simulink model "Channelizer_hil"  (R2023b)
settings: Solver=VariableStepAuto  StartTime=0.0  StopTime=inf  RelTol=1e-3
InitFcn:
  | init
values from neighbouring files (symbols this model uses):
  N = 2*1024    (= 2048)    [hil.m]    (also in init.m)
undefined symbols (not defined in the file or in its folder): ch0, ch1, ch10, ch11, ch12, ch13, ch14, ch15, ch2, ch3, ch4, ch5, ch6, ch7, ch8, ch9, S, vsva2197, xcvc1902
libraries: aieUtilities x47, aieBasic x34, hlsBasic x3, dspindex x3, vmcUtilities x1, commchan3 x1, commrflib2 x1, commfilt2 x1, commrandsrc3 x1, commdigbbndam3 x1
(part 2 of 2)

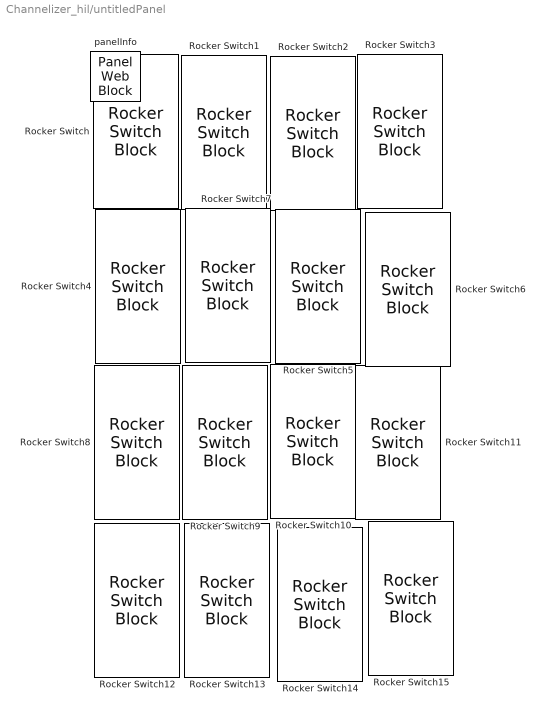
== system Channelizer_hil/untitledPanel ==
  Rocker Switch : RockerSwitchBlock  Tag=HiddenForWebPanel  PanelInfo="{\"addnFilesFolder\":\"\",\"height\":154,\"includeDebugPackages\":false,\"left\":10,\"outputFolder\":\"\",\"panelId\":\"panelId-fec1c322-f5e7-4e4f-8c31-b98d6132c1cd\",\"popoutMode\":\"\",\"standaloneTitle\":\"\",\"top\":12,\"type\":\"panelChild\",\"version\":\"2019b\",\"width\":85,\"zIndex\":1500002}"
      settings: Values={{'Off', 'On'}, [0 1]}
  Rocker Switch1 : RockerSwitchBlock  Tag=HiddenForWebPanel  PanelInfo="{\"addnFilesFolder\":\"\",\"height\":154,\"includeDebugPackages\":false,\"left\":98,\"outputFolder\":\"\",\"panelId\":\"panelId-fec1c322-f5e7-4e4f-8c31-b98d6132c1cd\",\"popoutMode\":\"\",\"standaloneTitle\":\"\",\"top\":12,\"type\":\"panelChild\",\"version\":\"2019b\",\"width\":85,\"zIndex\":1500004}"
      settings: Values={{'Off', 'On'}, [0 1]}
  Rocker Switch10 : RockerSwitchBlock  Tag=HiddenForWebPanel  PanelInfo="{\"addnFilesFolder\":\"\",\"height\":154,\"includeDebugPackages\":false,\"left\":185,\"outputFolder\":\"\",\"panelId\":\"panelId-fec1c322-f5e7-4e4f-8c31-b98d6132c1cd\",\"popoutMode\":\"\",\"standaloneTitle\":\"\",\"top\":327,\"type\":\"panelChild\",\"version\":\"2019b\",\"width\":85,\"zIndex\":1500022}"
      settings: Values={{'Off', 'On'}, [0 1]}
  Rocker Switch11 : RockerSwitchBlock  Tag=HiddenForWebPanel  PanelInfo="{\"addnFilesFolder\":\"\",\"height\":154,\"includeDebugPackages\":false,\"left\":273,\"outputFolder\":\"\",\"panelId\":\"panelId-fec1c322-f5e7-4e4f-8c31-b98d6132c1cd\",\"popoutMode\":\"\",\"standaloneTitle\":\"\",\"top\":327,\"type\":\"panelChild\",\"version\":\"2019b\",\"width\":85,\"zIndex\":1500024}"
      settings: Values={{'Off', 'On'}, [0 1]}
  Rocker Switch12 : RockerSwitchBlock  Tag=HiddenForWebPanel  PanelInfo="{\"addnFilesFolder\":\"\",\"height\":154,\"includeDebugPackages\":false,\"left\":10,\"outputFolder\":\"\",\"panelId\":\"panelId-fec1c322-f5e7-4e4f-8c31-b98d6132c1cd\",\"popoutMode\":\"\",\"standaloneTitle\":\"\",\"top\":483,\"type\":\"panelChild\",\"version\":\"2019b\",\"width\":85,\"zIndex\":1500026}"
      settings: Values={{'Off', 'On'}, [0 1]}
  Rocker Switch13 : RockerSwitchBlock  Tag=HiddenForWebPanel  PanelInfo="{\"addnFilesFolder\":\"\",\"height\":154,\"includeDebugPackages\":false,\"left\":97,\"outputFolder\":\"\",\"panelId\":\"panelId-fec1c322-f5e7-4e4f-8c31-b98d6132c1cd\",\"popoutMode\":\"\",\"standaloneTitle\":\"\",\"top\":483,\"type\":\"panelChild\",\"version\":\"2019b\",\"width\":85,\"zIndex\":1500028}"
      settings: Values={{'Off', 'On'}, [0 1]}
  Rocker Switch14 : RockerSwitchBlock  Tag=HiddenForWebPanel  PanelInfo="{\"addnFilesFolder\":\"\",\"height\":154,\"includeDebugPackages\":false,\"left\":185,\"outputFolder\":\"\",\"panelId\":\"panelId-fec1c322-f5e7-4e4f-8c31-b98d6132c1cd\",\"popoutMode\":\"\",\"standaloneTitle\":\"\",\"top\":484,\"type\":\"panelChild\",\"version\":\"2019b\",\"width\":85,\"zIndex\":1500030}"
      settings: Values={{'Off', 'On'}, [0 1]}
  Rocker Switch15 : RockerSwitchBlock  Tag=HiddenForWebPanel  PanelInfo="{\"addnFilesFolder\":\"\",\"height\":154,\"includeDebugPackages\":false,\"left\":272,\"outputFolder\":\"\",\"panelId\":\"panelId-fec1c322-f5e7-4e4f-8c31-b98d6132c1cd\",\"popoutMode\":\"\",\"standaloneTitle\":\"\",\"top\":484,\"type\":\"panelChild\",\"version\":\"2019b\",\"width\":85,\"zIndex\":1500032}"
      settings: Values={{'Off', 'On'}, [0 1]}
  Rocker Switch2 : RockerSwitchBlock  Tag=HiddenForWebPanel  PanelInfo="{\"addnFilesFolder\":\"\",\"height\":154,\"includeDebugPackages\":false,\"left\":186,\"outputFolder\":\"\",\"panelId\":\"panelId-fec1c322-f5e7-4e4f-8c31-b98d6132c1cd\",\"popoutMode\":\"\",\"standaloneTitle\":\"\",\"top\":12,\"type\":\"panelChild\",\"version\":\"2019b\",\"width\":85,\"zIndex\":1500006}"
      settings: Values={{'Off', 'On'}, [0 1]}
  Rocker Switch3 : RockerSwitchBlock  Tag=HiddenForWebPanel  PanelInfo="{\"addnFilesFolder\":\"\",\"height\":154,\"includeDebugPackages\":false,\"left\":274,\"outputFolder\":\"\",\"panelId\":\"panelId-fec1c322-f5e7-4e4f-8c31-b98d6132c1cd\",\"popoutMode\":\"\",\"standaloneTitle\":\"\",\"top\":12,\"type\":\"panelChild\",\"version\":\"2019b\",\"width\":85,\"zIndex\":1500008}"
      settings: Values={{'Off', 'On'}, [0 1]}
  Rocker Switch4 : RockerSwitchBlock  Tag=HiddenForWebPanel  PanelInfo="{\"addnFilesFolder\":\"\",\"height\":154,\"includeDebugPackages\":false,\"left\":10,\"outputFolder\":\"\",\"panelId\":\"panelId-fec1c322-f5e7-4e4f-8c31-b98d6132c1cd\",\"popoutMode\":\"\",\"standaloneTitle\":\"\",\"top\":169,\"type\":\"panelChild\",\"version\":\"2019b\",\"width\":85,\"zIndex\":1500010}"
      settings: Values={{'Off', 'On'}, [0 1]}
  Rocker Switch5 : RockerSwitchBlock  Tag=HiddenForWebPanel  PanelInfo="{\"addnFilesFolder\":\"\",\"height\":154,\"includeDebugPackages\":false,\"left\":186,\"outputFolder\":\"\",\"panelId\":\"panelId-fec1c322-f5e7-4e4f-8c31-b98d6132c1cd\",\"popoutMode\":\"\",\"standaloneTitle\":\"\",\"top\":170,\"type\":\"panelChild\",\"version\":\"2019b\",\"width\":85,\"zIndex\":1500012}"
      settings: Values={{'Off', 'On'}, [0 1]}
  Rocker Switch6 : RockerSwitchBlock  Tag=HiddenForWebPanel  PanelInfo="{\"addnFilesFolder\":\"\",\"height\":154,\"includeDebugPackages\":false,\"left\":274,\"outputFolder\":\"\",\"panelId\":\"panelId-fec1c322-f5e7-4e4f-8c31-b98d6132c1cd\",\"popoutMode\":\"\",\"standaloneTitle\":\"\",\"top\":170,\"type\":\"panelChild\",\"version\":\"2019b\",\"width\":85,\"zIndex\":1500014}"
      settings: Values={{'Off', 'On'}, [0 1]}
  Rocker Switch7 : RockerSwitchBlock  Tag=HiddenForWebPanel  PanelInfo="{\"addnFilesFolder\":\"\",\"height\":154,\"includeDebugPackages\":false,\"left\":98,\"outputFolder\":\"\",\"panelId\":\"panelId-fec1c322-f5e7-4e4f-8c31-b98d6132c1cd\",\"popoutMode\":\"\",\"standaloneTitle\":\"\",\"top\":169,\"type\":\"panelChild\",\"version\":\"2019b\",\"width\":85,\"zIndex\":1500016}"
      settings: Values={{'Off', 'On'}, [0 1]}
  Rocker Switch8 : RockerSwitchBlock  Tag=HiddenForWebPanel  PanelInfo="{\"addnFilesFolder\":\"\",\"height\":154,\"includeDebugPackages\":false,\"left\":10,\"outputFolder\":\"\",\"panelId\":\"panelId-fec1c322-f5e7-4e4f-8c31-b98d6132c1cd\",\"popoutMode\":\"\",\"standaloneTitle\":\"\",\"top\":326,\"type\":\"panelChild\",\"version\":\"2019b\",\"width\":85,\"zIndex\":1500018}"
      settings: Values={{'Off', 'On'}, [0 1]}
  Rocker Switch9 : RockerSwitchBlock  Tag=HiddenForWebPanel  PanelInfo="{\"addnFilesFolder\":\"\",\"height\":154,\"includeDebugPackages\":false,\"left\":97,\"outputFolder\":\"\",\"panelId\":\"panelId-fec1c322-f5e7-4e4f-8c31-b98d6132c1cd\",\"popoutMode\":\"\",\"standaloneTitle\":\"\",\"top\":326,\"type\":\"panelChild\",\"version\":\"2019b\",\"width\":85,\"zIndex\":1500020}"
      settings: Values={{'Off', 'On'}, [0 1]}
  panelInfo : PanelWebBlock  Tag=HiddenForWebPanel  PanelInfo="{\"addnFilesFolder\":\"\",\"compacted\":false,\"height\":655,\"includeDebugPackages\":false,\"isActiveTab\":true,\"left\":-4,\"name\":\"Panel\",\"outputFolder\":\"\",\"panelId\":\"panelId-fec1c322-f5e7-4e4f-8c31-b98d6132c1cd\",\"popoutMode\":\"\",\"standaloneTitle\":\"\",\"tabIndex\":0,\"tabbedSetId\":\"tabbedSet6868322055\",\"top\":96,\"type\":\"panel\",\"version\":\"2019b\",\"visible\":true,\"width\":371,\"zIndex\":1500002}"  PanelSnapshot=<binary blob, 10492 chars, not shown>

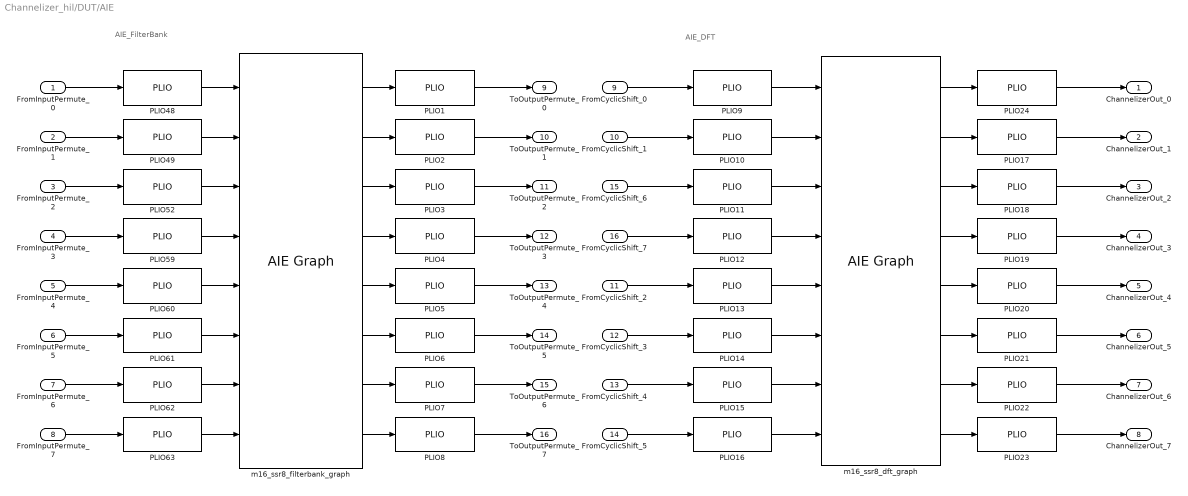
== system Channelizer_hil/DUT/AIE ==
  note: AIE_DFT
  note: AIE_FilterBank
  FromInputPermute_0 : Inport
  FromInputPermute_1 : Inport  Port=2
  FromInputPermute_2 : Inport  Port=3
  FromInputPermute_3 : Inport  Port=4
  FromInputPermute_4 : Inport  Port=5
  FromInputPermute_5 : Inport  Port=6
  FromInputPermute_6 : Inport  Port=7
  FromInputPermute_7 : Inport  Port=8
  FromCyclicShift_0 : Inport  Port=9
  FromCyclicShift_1 : Inport  Port=10
  FromCyclicShift_2 : Inport  Port=11
  FromCyclicShift_3 : Inport  Port=12
  FromCyclicShift_4 : Inport  Port=13
  FromCyclicShift_5 : Inport  Port=14
  FromCyclicShift_6 : Inport  Port=15
  FromCyclicShift_7 : Inport  Port=16
  PLIO{1..24,48..49,52,59..63} (32 alike) : aieBasic/PLIO  PlioWidth=64  PlioFreqSpec=on  PlioFreq=625  ColLocation=0  channel=0  blockJsonConstraints=[]  deprecateConstraints=0
  m16_ssr8_dft_graph : aieBasic/AIE Graph  PortAttributesTable={ 'Input', 'sig_i[0]', 'stream', 'cint16', '', '', ''; 'Input', 'sig_i[1]', 'stream', 'cint16', '', '', ''; 'Input', 'sig_i[6]', 'stream', 'cint16', '', '', ''; 'Input', 'sig_i[7]', 'stream', 'cint16', '', '', ''; 'Input', 'sig_i[2]', 'stream', 'cint16', '', '', ''; 'Input', 'sig_i[3]', 'stream', 'cint16', '', '', ''; 'Input', 'sig_i[4]', 'stream', 'cint16', '', '', ''; 'Input', 'sig_i[5]', 'stream', 'cint16', '', '', ''; 'Output', 'sig_o[0]', 'stream', 'cint16', '', '', '4*N'; 'Output', 'sig_o[1]', 'stream', 'cint16', '', '', '4*N'; 'Output', 'sig_o[2]', 'stream', 'cint16', '', '', '4*N'; 'Output', 'sig_o[3]', 'stream', 'cint16', '', '', '4*N'; 'Output', 'sig_o[4]', 'stream', 'cint16', '', '', '4*N'; 'Output', 'sig_o[5]', 'stream', 'cint16', '', '', '4*N'; 'Output', 'sig_o[6]', 'stream', 'cint16', '', '', '4*N'; 'Output', 'sig_o[7]', 'stream', 'cint16', '', '', '4*N' }  PortAttributesEnablement={'off', 'on', 'off', 'off', 'off', 'off', 'off';'off', 'on', 'off', 'off', 'off', 'off', 'off';'off', 'on', 'off', 'off', 'off', 'off', 'off';'off', 'on', 'off', 'off', 'off', 'off', 'off';'off', 'on', 'off', 'off', 'off', 'off', 'off';'off', 'on', 'off', 'off', 'off', 'off', 'off';'off', 'on', 'off', 'off', 'off', 'off', 'off';'off', 'on', 'off', 'off', 'off', 'off', 'off';'off', 'on', 'off', 'off', 'off', 'off', 'on';'off', 'on', 'off', 'off', 'off', 'off', 'on';'off', 'on', 'off', 'off', 'off', 'off', 'on';'off', 'on', 'off', 'off', 'off', 'off', 'on';'off', 'on', 'off', 'off', 'off', 'off', 'on';'off', 'on', 'off', 'off', 'off', 'off', 'on';'off', 'on', 'off', 'off', 'off', 'off', 'on';'off', 'on', 'off', 'off', 'off', 'off', 'on'}  SampleTime=-1  ClassDeclTypeOptions=C[1 1]@t24@class m16_ssr8_dft_graph  ClassDecl=class m16_ssr8_dft_graph  ClassTemplateParams={}  ClassTemplateParamsEnables={}  ClassCtorDeclTypeOptions=C[1 1]@t7@<empty>  ClassCtorDecl=<empty>  ClassCtorParams={}  GraphAllAttrs=|  PortArgDecls={'in stream cint16 in1'; 'in stream cint16 in2'; 'in stream cint16 in3'; 'in stream cint16 in4'; 'in stream cint16 in5'; 'in stream cint16 in6'; 'in stream cint16 in7'; 'in stream cint16 in8'; 'out stream cint16 out1'; 'out stream cint16 out2'; 'out stream cint16 out3'; 'out stream cint16 out4'; 'out stream cint16 out5'; 'out stream cint16 out6'; 'out stream cint16 out7'; 'out stream cint16 out8'}  PortGraphPortNames={'sig_i[0]'; 'sig_i[1]'; 'sig_i[6]'; 'sig_i[7]'; 'sig_i[2]'; 'sig_i[3]'; 'sig_i[4]'; 'sig_i[5]'; 'sig_o[0]'; 'sig_o[1]'; 'sig_o[2]'; 'sig_o[3]'; 'sig_o[4]'; 'sig_o[5]'; 'sig_o[6]'; 'sig_o[7]'}  PortTypes={'stream'; 'stream'; 'stream'; 'stream'; 'stream'; 'stream'; 'stream'; 'stream'; 'stream'; 'stream'; 'stream'; 'stream'; 'stream'; 'stream'; 'stream'; 'stream'}  PortDataTypes={'cint16'; 'cint16'; 'cint16'; 'cint16'; 'cint16'; 'cint16'; 'cint16'; 'cint16'; 'cint16'; 'cint16'; 'cint16'; 'cint16'; 'cint16'; 'cint16'; 'cint16'; 'cint16'}  PortSizes={0.000000000000000000e+00; 0.000000000000000000e+00; 0.000000000000000000e+00; 0.000000000000000000e+00; 0.000000000000000000e+00; 0.000000000000000000e+00; 0.000000000000000000e+00; 0.000000000000000000e+00; 0.000000000000000000e+00; 0.000000000000000000e+00; 0.000000000000000000e+00; 0.000000000000000000e+00; 0.000000000000000000e+00; 0.000000000000000000e+00; 0.000000000000000000e+00; 0.000000000000000000e+00}  PortSynchronicities={'auto'; 'auto'; 'auto'; 'auto'; 'auto'; 'auto'; 'auto'; 'auto'; 'auto'; 'auto'; 'auto'; 'auto'; 'auto'; 'auto'; 'auto'; 'auto'}  PortSignalSizes={0.000000000000000000e+00; 0.000000000000000000e+00; 0.000000000000000000e+00; 0.000000000000000000e+00; 0.000000000000000000e+00; 0.000000000000000000e+00; 0.000000000000000000e+00; 0.000000000000000000e+00; 8.192000000000000000e+03; 8.192000000000000000e+03; 8.192000000000000000e+03; 8.192000000000000000e+03; 8.192000000000000000e+03; 8.192000000000000000e+03; 8.192000000000000000e+03; 8.192000000000000000e+03}  SimLibPath=''  ClassIndex=1  ClassCtorIndex=0  ClassTabVisible=off  FunctionTabVisible=on  DelayDrawLabels=off  GraphFileSelect=Header file (*.h)  GraphHeaderFile=./aie/m16_ssr8_dft_graph.h  GraphClassName=m16_ssr8_dft_graph  GraphName=m16_ssr8_dft_graph  GraphHeaderFiles={'./aie/dft_1xN_widget_graph.h'; './aie/m16_ssr8_dft_graph.h'}  GraphSourceFile=./model_composer_work/xmc_aie_lib/8d40d72d/mygraph.cpp  GraphSearchPaths={'./aie'}  GraphPreProcOptions={}  blockJsonConstraints=[]
      | s[12;12;9;9;19;14;21;23;21;23;24;21;15;17;12;24;26;26;26;27;28;9;21;23;23;23;24;25;14;19;19;29]@FunctionNameDeclFileNamePortNamesPortTypesPortSerializedTypesPortDirectionsPortWindowSizeEnablesPortWindowMarginEnablesPortBufferSizeEnablesPortBufferMarginEnablesPortSynchronicityEnablesPortSignalSizeEnablesPortBufferSizesPortBufferMarginsFunctionDeclFunctionTemplateSpecKindFunctionTemplateParamNamesFunctionTemplateParamKindsFunctionTemplateParamTypesFunctionTemplateParamValuesFunctionTemplateParamEnablesClassDeclClassTemplateSpecKindClassTemplateParamNamesClassTemplateParamKindsClassTemplateParamTypesClassTemplateParamValuesClassTemplateParamEnablesClassCtorDeclsClassCtorParamNamesClassCtorParamTypesClassCtorParamSerializedTypes[1 1]@C[32 1]@nt30@../../aie/m16_ssr8_dft_graph.hC[2 1]@t5@sig_it5@sig_oC[2 1]@t48@std::array< adf::port< adf::direction::in >, 8 >t49@std::array< adf::port< adf::direction::out >, 8 >C[2 1]@t64@{Tstd::array{2{t{Tadf::port{1{t{Sadf::direction::in}}}}}{t{}8}}}t65@{Tstd::array{2{t{Tadf::port{1{t{Sadf::direction::out}}}}}{t{}8}}}C[2 1]@t5@inputt5@inputC[2 1]@l0@l0@C[2 1]@l0@l0@C[2 1]@l0@l0@C[2 1]@l0@l0@C[2 1]@l1@l1@C[2 1]@l0@l0@C[2 1]@nnC[2 1]@nnt139@void m16_ssr8_dft_graph::
      | (std::array< adf::port< adf::direction::in >, 8 > sig_i, std::array< adf::port< adf::direction::out >, 8 > sig_o)ne[0 1]@e[0 1]@e[0 1]@e[0 1]@e[0 1]@t25@class m16_ssr8_dft_graph;t4@nonee[0 1]@e[0 1]@e[0 1]@e[0 1]@e[0 1]@e[0 1]@e[0 1]@e[0 1]@e[0 1]@
  m16_ssr8_filterbank_graph : aieBasic/AIE Graph  PortAttributesTable={ 'Input', 'sig_i[0]', 'stream', 'cint16', '', '', ''; 'Input', 'sig_i[1]', 'stream', 'cint16', '', '', ''; 'Input', 'sig_i[2]', 'stream', 'cint16', '', '', ''; 'Input', 'sig_i[3]', 'stream', 'cint16', '', '', ''; 'Input', 'sig_i[4]', 'stream', 'cint16', '', '', ''; 'Input', 'sig_i[5]', 'stream', 'cint16', '', '', ''; 'Input', 'sig_i[6]', 'stream', 'cint16', '', '', ''; 'Input', 'sig_i[7]', 'stream', 'cint16', '', '', ''; 'Output', 'sig_o[0]', 'stream', 'cint16', '', '', '4*N'; 'Output', 'sig_o[1]', 'stream', 'cint16', '', '', '4*N'; 'Output', 'sig_o[2]', 'stream', 'cint16', '', '', '4*N'; 'Output', 'sig_o[3]', 'stream', 'cint16', '', '', '4*N'; 'Output', 'sig_o[4]', 'stream', 'cint16', '', '', '4*N'; 'Output', 'sig_o[5]', 'stream', 'cint16', '', '', '4*N'; 'Output', 'sig_o[6]', 'stream', 'cint16', '', '', '4*N'; 'Output', 'sig_o[7]', 'stream', 'cint16', '', '', '4*N' }  PortAttributesEnablement={'off', 'on', 'off', 'off', 'off', 'off', 'off';'off', 'on', 'off', 'off', 'off', 'off', 'off';'off', 'on', 'off', 'off', 'off', 'off', 'off';'off', 'on', 'off', 'off', 'off', 'off', 'off';'off', 'on', 'off', 'off', 'off', 'off', 'off';'off', 'on', 'off', 'off', 'off', 'off', 'off';'off', 'on', 'off', 'off', 'off', 'off', 'off';'off', 'on', 'off', 'off', 'off', 'off', 'off';'off', 'on', 'off', 'off', 'off', 'off', 'on';'off', 'on', 'off', 'off', 'off', 'off', 'on';'off', 'on', 'off', 'off', 'off', 'off', 'on';'off', 'on', 'off', 'off', 'off', 'off', 'on';'off', 'on', 'off', 'off', 'off', 'off', 'on';'off', 'on', 'off', 'off', 'off', 'off', 'on';'off', 'on', 'off', 'off', 'off', 'off', 'on';'off', 'on', 'off', 'off', 'off', 'off', 'on'}  SampleTime=-1  ClassDeclTypeOptions=C[1 1]@t31@class m16_ssr8_filterbank_graph  ClassDecl=class m16_ssr8_filterbank_graph  ClassTemplateParams={}  ClassTemplateParamsEnables={}  ClassCtorDeclTypeOptions=C[1 1]@t7@<empty>  ClassCtorDecl=<empty>  ClassCtorParams={}  GraphAllAttrs=|  PortArgDecls={'in stream cint16 in1'; 'in stream cint16 in2'; 'in stream cint16 in3'; 'in stream cint16 in4'; 'in stream cint16 in5'; 'in stream cint16 in6'; 'in stream cint16 in7'; 'in stream cint16 in8'; 'out stream cint16 out1'; 'out stream cint16 out2'; 'out stream cint16 out3'; 'out stream cint16 out4'; 'out stream cint16 out5'; 'out stream cint16 out6'; 'out stream cint16 out7'; 'out stream cint16 out8'}  PortGraphPortNames={'sig_i[0]'; 'sig_i[1]'; 'sig_i[2]'; 'sig_i[3]'; 'sig_i[4]'; 'sig_i[5]'; 'sig_i[6]'; 'sig_i[7]'; 'sig_o[0]'; 'sig_o[1]'; 'sig_o[2]'; 'sig_o[3]'; 'sig_o[4]'; 'sig_o[5]'; 'sig_o[6]'; 'sig_o[7]'}  PortTypes={'stream'; 'stream'; 'stream'; 'stream'; 'stream'; 'stream'; 'stream'; 'stream'; 'stream'; 'stream'; 'stream'; 'stream'; 'stream'; 'stream'; 'stream'; 'stream'}  PortDataTypes={'cint16'; 'cint16'; 'cint16'; 'cint16'; 'cint16'; 'cint16'; 'cint16'; 'cint16'; 'cint16'; 'cint16'; 'cint16'; 'cint16'; 'cint16'; 'cint16'; 'cint16'; 'cint16'}  PortSizes={0.000000000000000000e+00; 0.000000000000000000e+00; 0.000000000000000000e+00; 0.000000000000000000e+00; 0.000000000000000000e+00; 0.000000000000000000e+00; 0.000000000000000000e+00; 0.000000000000000000e+00; 0.000000000000000000e+00; 0.000000000000000000e+00; 0.000000000000000000e+00; 0.000000000000000000e+00; 0.000000000000000000e+00; 0.000000000000000000e+00; 0.000000000000000000e+00; 0.000000000000000000e+00}  PortSynchronicities={'auto'; 'auto'; 'auto'; 'auto'; 'auto'; 'auto'; 'auto'; 'auto'; 'auto'; 'auto'; 'auto'; 'auto'; 'auto'; 'auto'; 'auto'; 'auto'}  PortSignalSizes={0.000000000000000000e+00; 0.000000000000000000e+00; 0.000000000000000000e+00; 0.000000000000000000e+00; 0.000000000000000000e+00; 0.000000000000000000e+00; 0.000000000000000000e+00; 0.000000000000000000e+00; 8.192000000000000000e+03; 8.192000000000000000e+03; 8.192000000000000000e+03; 8.192000000000000000e+03; 8.192000000000000000e+03; 8.192000000000000000e+03; 8.192000000000000000e+03; 8.192000000000000000e+03}  SimLibPath=''  ClassIndex=1  ClassCtorIndex=0  ClassTabVisible=off  FunctionTabVisible=on  DelayDrawLabels=off  GraphFileSelect=Header file (*.h)  GraphHeaderFile=./aie/m16_ssr8_filterbank_graph.h  GraphClassName=m16_ssr8_filterbank_graph  GraphName=m16_ssr8_filterbank_graph  GraphHeaderFiles={'./aie/polyphase_fir_graph.h'; './aie/m16_ssr8_filterbank_graph.h'}  GraphSourceFile=./model_composer_work/xmc_aie_lib/fadd8e47/mygraph.cpp  GraphSearchPaths={'./aie'}  GraphPreProcOptions={}  blockJsonConstraints=[]
      | s[12;12;9;9;19;14;21;23;21;23;24;21;15;17;12;24;26;26;26;27;28;9;21;23;23;23;24;25;14;19;19;29]@FunctionNameDeclFileNamePortNamesPortTypesPortSerializedTypesPortDirectionsPortWindowSizeEnablesPortWindowMarginEnablesPortBufferSizeEnablesPortBufferMarginEnablesPortSynchronicityEnablesPortSignalSizeEnablesPortBufferSizesPortBufferMarginsFunctionDeclFunctionTemplateSpecKindFunctionTemplateParamNamesFunctionTemplateParamKindsFunctionTemplateParamTypesFunctionTemplateParamValuesFunctionTemplateParamEnablesClassDeclClassTemplateSpecKindClassTemplateParamNamesClassTemplateParamKindsClassTemplateParamTypesClassTemplateParamValuesClassTemplateParamEnablesClassCtorDeclsClassCtorParamNamesClassCtorParamTypesClassCtorParamSerializedTypes[1 1]@C[32 1]@nt37@../../aie/m16_ssr8_filterbank_graph.hC[2 1]@t5@sig_it5@sig_oC[2 1]@t48@std::array< adf::port< adf::direction::in >, 8 >t49@std::array< adf::port< adf::direction::out >, 8 >C[2 1]@t64@{Tstd::array{2{t{Tadf::port{1{t{Sadf::direction::in}}}}}{t{}8}}}t65@{Tstd::array{2{t{Tadf::port{1{t{Sadf::direction::out}}}}}{t{}8}}}C[2 1]@t5@inputt5@inputC[2 1]@l0@l0@C[2 1]@l0@l0@C[2 1]@l0@l0@C[2 1]@l0@l0@C[2 1]@l1@l1@C[2 1]@l0@l0@C[2 1]@nnC[2 1]@nnt146@void m16_ssr8_filterbank_graph::
      | (std::array< adf::port< adf::direction::in >, 8 > sig_i, std::array< adf::port< adf::direction::out >, 8 > sig_o)ne[0 1]@e[0 1]@e[0 1]@e[0 1]@e[0 1]@t32@class m16_ssr8_filterbank_graph;t4@nonee[0 1]@e[0 1]@e[0 1]@e[0 1]@e[0 1]@e[0 1]@e[0 1]@e[0 1]@e[0 1]@
  ChannelizerOut_0 : Outport
  ChannelizerOut_1 : Outport  Port=2
  ChannelizerOut_2 : Outport  Port=3
  ChannelizerOut_3 : Outport  Port=4
  ChannelizerOut_4 : Outport  Port=5
  ChannelizerOut_5 : Outport  Port=6
  ChannelizerOut_6 : Outport  Port=7
  ChannelizerOut_7 : Outport  Port=8
  ToOutputPermute_0 : Outport  Port=9
  ToOutputPermute_1 : Outport  Port=10
  ToOutputPermute_2 : Outport  Port=11
  ToOutputPermute_3 : Outport  Port=12
  ToOutputPermute_4 : Outport  Port=13
  ToOutputPermute_5 : Outport  Port=14
  ToOutputPermute_6 : Outport  Port=15
  ToOutputPermute_7 : Outport  Port=16
  wires:
  PLIO4/1 -> ToOutputPermute_3/1
  PLIO1/1 -> ToOutputPermute_0/1
  PLIO2/1 -> ToOutputPermute_1/1
  PLIO8/1 -> ToOutputPermute_7/1
  PLIO7/1 -> ToOutputPermute_6/1
  PLIO5/1 -> ToOutputPermute_4/1
  PLIO6/1 -> ToOutputPermute_5/1
  PLIO3/1 -> ToOutputPermute_2/1
  PLIO22/1 -> ChannelizerOut_6/1
  PLIO21/1 -> ChannelizerOut_5/1
  PLIO24/1 -> ChannelizerOut_0/1
  PLIO17/1 -> ChannelizerOut_1/1
  PLIO18/1 -> ChannelizerOut_2/1
  PLIO19/1 -> ChannelizerOut_3/1
  PLIO20/1 -> ChannelizerOut_4/1
  PLIO23/1 -> ChannelizerOut_7/1
  m16_ssr8_filterbank_graph/1 -> PLIO1/1
  m16_ssr8_filterbank_graph/7 -> PLIO7/1
  m16_ssr8_filterbank_graph/6 -> PLIO6/1
  PLIO59/1 -> m16_ssr8_filterbank_graph/4
  PLIO63/1 -> m16_ssr8_filterbank_graph/8
  FromInputPermute_0/1 -> PLIO48/1
  FromInputPermute_4/1 -> PLIO60/1
  PLIO61/1 -> m16_ssr8_filterbank_graph/6
  FromInputPermute_2/1 -> PLIO52/1
  PLIO52/1 -> m16_ssr8_filterbank_graph/3
  FromInputPermute_6/1 -> PLIO62/1
  FromInputPermute_5/1 -> PLIO61/1
  PLIO62/1 -> m16_ssr8_filterbank_graph/7
  FromInputPermute_3/1 -> PLIO59/1
  m16_ssr8_filterbank_graph/5 -> PLIO5/1
  FromInputPermute_7/1 -> PLIO63/1
  PLIO49/1 -> m16_ssr8_filterbank_graph/2
  m16_ssr8_filterbank_graph/8 -> PLIO8/1
  FromInputPermute_1/1 -> PLIO49/1
  PLIO60/1 -> m16_ssr8_filterbank_graph/5
  m16_ssr8_filterbank_graph/3 -> PLIO3/1
  PLIO48/1 -> m16_ssr8_filterbank_graph/1
  m16_ssr8_filterbank_graph/2 -> PLIO2/1
  m16_ssr8_filterbank_graph/4 -> PLIO4/1
  FromCyclicShift_3/1 -> PLIO14/1
  PLIO13/1 -> m16_ssr8_dft_graph/5
  m16_ssr8_dft_graph/8 -> PLIO23/1
  PLIO16/1 -> m16_ssr8_dft_graph/8
  FromCyclicShift_5/1 -> PLIO16/1
  m16_ssr8_dft_graph/1 -> PLIO24/1
  FromCyclicShift_2/1 -> PLIO13/1
  m16_ssr8_dft_graph/3 -> PLIO18/1
  FromCyclicShift_1/1 -> PLIO10/1
  m16_ssr8_dft_graph/6 -> PLIO21/1
  m16_ssr8_dft_graph/5 -> PLIO20/1
  PLIO12/1 -> m16_ssr8_dft_graph/4
  FromCyclicShift_7/1 -> PLIO12/1
  FromCyclicShift_6/1 -> PLIO11/1
  m16_ssr8_dft_graph/2 -> PLIO17/1
  FromCyclicShift_0/1 -> PLIO9/1
  PLIO10/1 -> m16_ssr8_dft_graph/2
  PLIO11/1 -> m16_ssr8_dft_graph/3
  PLIO9/1 -> m16_ssr8_dft_graph/1
  PLIO15/1 -> m16_ssr8_dft_graph/7
  FromCyclicShift_4/1 -> PLIO15/1
  m16_ssr8_dft_graph/4 -> PLIO19/1
  PLIO14/1 -> m16_ssr8_dft_graph/6
  m16_ssr8_dft_graph/7 -> PLIO22/1
